simulink model "DinamicaTesis"  (R2021b)
settings: Solver=VariableStepAuto  StartTime=0.0  StopTime=50  RelTol=1e-3
(part 3 of 3)

== matlab function DinamicaTesis/Embedded MATLAB Function3 ==
  data: q3 output; t input
function q3 = posq3(t)
% This block supports an embeddable subset of the MATLAB language.
% See the help menu for details. 

if (t>=17)  % Si el t>=tmax, se repite una vez la rutina
    t=t-17;
end

if(t<6) % Movimiento 1
    t_inic = 0; % Tiempo en que inicia
    tf = 4;     % Tiempo en que termina
    y_ini = 1.570;
    y_f = -0.785;
elseif (t>=6 && t<12) % Movimiento 2
    t_inic = 6;
    tf = 4;
    y_ini = -0.785;
    y_f = -0.785;
else  % Movimiento 3
    t_inic = 12;
    tf = 5;
    y_ini = -0.785;
    y_f =  1.570;
end

% Calculo de trayectoria de tiempo minimo
Tb = tf/2;
% Vmax = 2*(y_f - y_ini)/(tf);
Vmax = (y_f - y_ini)/(tf - Tb);
ta = t - t_inic;
if(ta<0)
    q3 = y_ini;
elseif(ta >= 0 && ta < Tb)
    q3 = y_ini + (Vmax/(2*Tb))*ta*ta;
elseif(ta >= Tb && ta < (tf - Tb))
    q3 = (y_ini + y_f - Vmax*tf)/2 + Vmax*ta;
elseif(ta >= (tf - Tb) && ta < tf)
     q3 = y_f - (Vmax*(tf-ta)*(tf-ta)/(2*Tb));
else
    q3 = y_f;
end
